simulink model "bias_nonZero_dotProduct"  (R2024b)
settings: Solver=FixedStepDiscrete  StartTime=0.0  StopTime=10.0  RelTol=1e-3
settings Model: Creator=optimus  LastModifiedBy=optimus

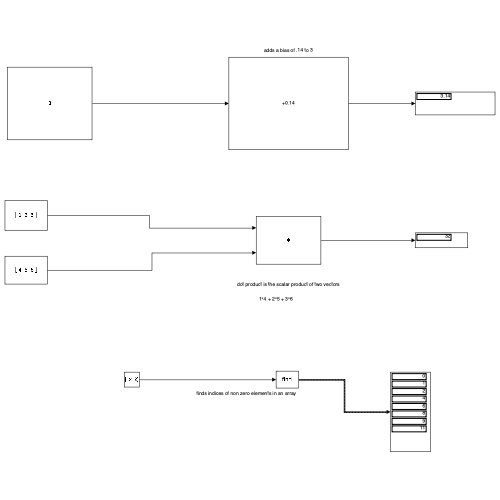
[thumbnail: Simulink's stored preview of the top-level diagram]
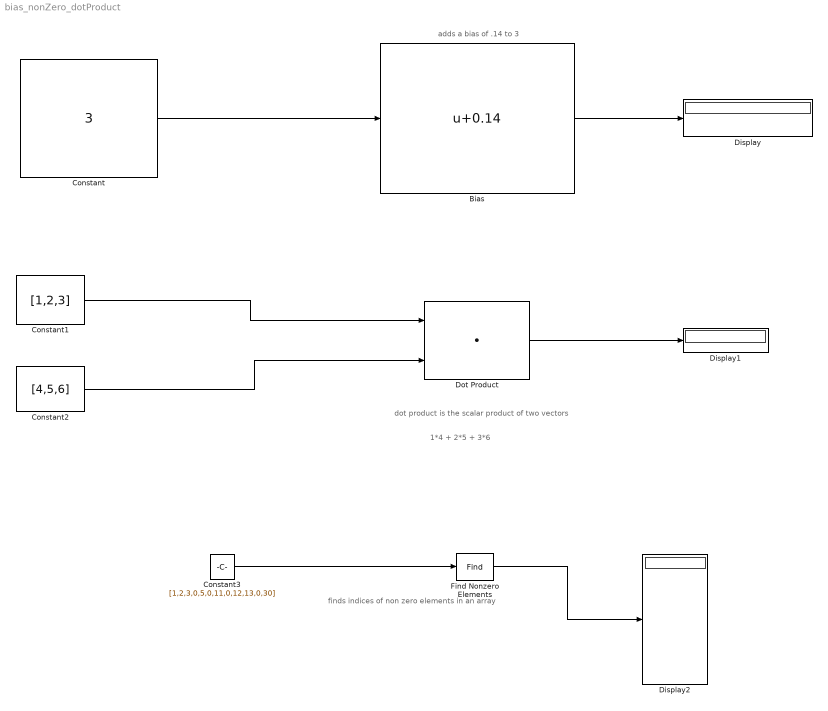
== system bias_nonZero_dotProduct ==
  note: finds indices of non zero elements in an array
  note: 1*4 + 2*5 + 3*6
  note: dot product is the scalar product of two vectors
  note: adds a bias of .14 to 3
  Bias : Bias  Bias=0.14  SaturateOnIntegerOverflow=off
  Constant : Constant  Value=3
  Constant1 : Constant  Value=[1,2,3]
  Constant2 : Constant  Value=[4,5,6]
  Constant3 : Constant  Value=[1,2,3,0,5,0,11,0,12,13,0,30]
  Display : Display
  Display1 : Display
  Display2 : Display
  Dot Product : DotProduct  OutDataTypeStr=Inherit: Inherit via internal rule
  Find Nonzero Elements : Find  NumberOfInputDimensions=3  IndexMode=Zero-based
  wires:
  Constant/1 -> Bias/1
  Bias/1 -> Display/1
  Constant1/1 -> Dot Product/1
  Constant2/1 -> Dot Product/2
  Dot Product/1 -> Display1/1
  Constant3/1 -> Find Nonzero Elements/1
  Find Nonzero Elements/1 -> Display2/1
